simulink model "h2omnix_manual"  (R2022b)
settings: Solver=ode4  StartTime=0.0  StopTime=inf  FixedStep=0.05  RelTol=1e-3
libraries: MarineRoboticsLibEx x1, MarineRoboticsLib x1
settings Model: DataDictionary=ros2lib.sldd  EnableAccessToBaseWorkspace=off  Creator=dnad  LastModifiedBy=dnad

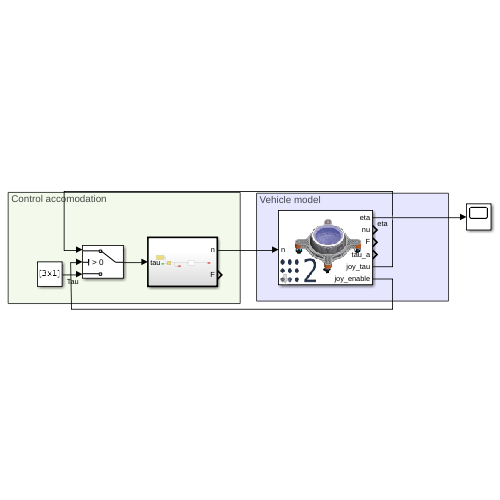
[thumbnail: Simulink's stored preview of the top-level diagram]
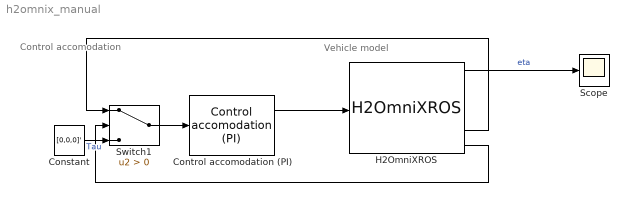
== system h2omnix_manual ==
  note: Control accomodation
  note: Vehicle model
  Constant : Constant  Value=[0,0,0]'
  Control accomodation (PI) : MarineRoboticsLibEx/Control accomodation (PI)  SystemSampleTime=-1  VariantActivationTime=update diagram  Latency=0  AutoFrameSizeCalculation=off
  H2OmniXROS : MarineRoboticsLib/H2OmniXROS  vehicle_name=krk  max_pwm=0.4  pwm_topic=/krk/pwm_out  odometry_topic=/krk/odometry/filtered  joy_topic=/krk/joy
  Scope : Scope
  Switch1 : Switch  Criteria=u2 > Threshold  SaturateOnIntegerOverflow=off  InputSameDT=off
  wires:
  Constant/1 -> Switch1/3  "Tau"
  Switch1/1 -> Control accomodation (PI)/1
  Control accomodation (PI)/1 -> H2OmniXROS/1
  H2OmniXROS/5 -> Switch1/1
  H2OmniXROS/6 -> Switch1/2
  H2OmniXROS/1 -> Scope/1  "eta"
